simulink model "Inversion"  (Simulink 7.9)
settings: Solver=ode45  StartTime=0.0  StopTime=8  RelTol=1e-3
values from neighbouring files (symbols this model uses):
  g = 9.81    [init.m]
  m = 1.863    [init.m]
undefined symbols (not defined in the file or in its folder): sigbuilder_block
settings Model: Creator=Matthias  LastModifiedBy=Matthias

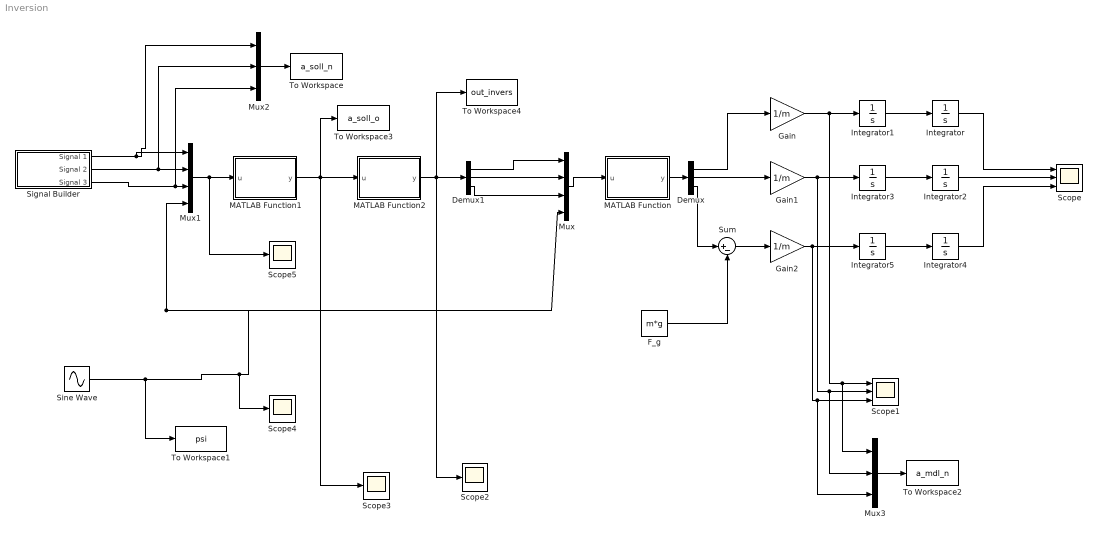
== system Inversion ==
  Demux : Demux  Outputs=3
  Demux1 : Demux  Outputs=3
  F_g : Constant  Value=m*g
  Gain : Gain  Gain=1/m
  Gain1 : Gain  Gain=1/m
  Gain2 : Gain  Gain=1/m
  Integrator{,1..5} (6 alike) : Integrator
  MATLAB Function : MATLAB Function  TreatAsAtomicUnit=on
  MATLAB Function1 : MATLAB Function  TreatAsAtomicUnit=on
  MATLAB Function2 : MATLAB Function  TreatAsAtomicUnit=on
  Mux : Mux
  Mux1 : Mux
  Mux2 : Mux  Inputs=3
  Mux3 : Mux  Inputs=3
  Scope : Scope  NumInputPorts=3
      settings: YMin=-5~-5~-5  YMax=5~5~5
  Scope1 : Scope  NumInputPorts=3
      settings: YMin=-5~-5~-5  YMax=5~5~5
  Scope{2..5} (4 alike) : Scope
      Scope2 settings: SaveName=ScopeData2
      Scope3 settings: SaveName=ScopeData3
      Scope4 settings: SaveName=ScopeData4
      Scope5 settings: SaveName=ScopeData5
  Signal Builder : Subsystem  Tag=STV Subsys  LoadFcn=sigbuilder_block('load',[403.5 141 550.5 395.25 ]);  StartFcn=sigbuilder_block('start');  StopFcn=sigbuilder_block('stop');  ClipboardFcn=sigbuilder_block('clipboard');  mask(Sigbuilder block){}
      mask help: Simulink:masks:SigbuilderBlock_MD
      mask init:
      | if ~strcmp(get_param(bdroot(gcbh),'SimulationStatus'),'stopped') tuvar = sigbuilder_block('maskInit'); end
      settings: CopyFcn=sigbuilder_block('copy');  DeleteFcn=sigbuilder_block('delete');  ModelCloseFcn=sigbuilder_block('modelClose');  PreSaveFcn=sigbuilder_block('preSave');  PauseFcn=sigbuilder_block('pause');  ContinueFcn=sigbuilder_block('continue');  NameChangeFcn=sigbuilder_block('namechange');  OpenFcn=sigbuilder_block('open',[437.6 199.2 550.4 400 ]);  CloseFcn=sigbuilder_block('close');
      mask Display: plot(0, 0, 100, 100,[2, 2, 32, 32, 2], [68, 8, 8, 68, 68],[32, 2], [38, 38], [32, 19, 2],[53, 60, 44], [32, 17, 17, 2],[16, 16, 31, 31]);txt = getActiveGroup(gcbh);text(2, 100, txt,'verticalAlignment', 'top');
  Sine Wave : Sin  SampleTime=0
  Sum : Sum  Inputs=|+-
  To Workspace : ToWorkspace  VariableName=a_soll_n  SampleTime=-1  SaveFormat=Structure With Time
  To Workspace1 : ToWorkspace  VariableName=psi  SampleTime=-1  SaveFormat=Structure With Time
  To Workspace2 : ToWorkspace  VariableName=a_mdl_n  SampleTime=-1  SaveFormat=Structure With Time
  To Workspace3 : ToWorkspace  VariableName=a_soll_o  SampleTime=-1  SaveFormat=Structure With Time
  To Workspace4 : ToWorkspace  VariableName=out_invers  SampleTime=-1  SaveFormat=Structure With Time
  wires:
  Integrator5/1 -> Integrator4/1
  Integrator3/1 -> Integrator2/1
  Integrator1/1 -> Integrator/1
  Integrator/1 -> Scope/1
  Integrator2/1 -> Scope/2
  Integrator4/1 -> Scope/3
  Gain/1 -> Integrator1/1, Scope1/1, Mux3/1
  Gain1/1 -> Integrator3/1, Scope1/2, Mux3/2
  Gain2/1 -> Integrator5/1, Scope1/3, Mux3/3
  Mux/1 -> MATLAB Function/1(u)
  MATLAB Function/1(y) -> Demux/1
  Demux/1 -> Gain/1
  Demux/2 -> Gain1/1
  Mux1/1 -> MATLAB Function1/1(u), Scope5/1
  Sine Wave/1 -> Mux1/4, Mux/4, Scope4/1, To Workspace1/1
  MATLAB Function1/1(y) -> MATLAB Function2/1(u), Scope3/1, To Workspace3/1
  MATLAB Function2/1(y) -> Demux1/1, Scope2/1, To Workspace4/1
  Demux1/1 -> Mux/1
  Demux1/2 -> Mux/2
  Demux1/3 -> Mux/3
  Demux/3 -> Sum/1
  F_g/1 -> Sum/2
  Sum/1 -> Gain2/1
  Signal Builder/1(Signal 1) -> Mux1/1, Mux2/1
  Signal Builder/2(Signal 2) -> Mux1/2, Mux2/2
  Signal Builder/3(Signal 3) -> Mux1/3, Mux2/3
  Mux2/1 -> To Workspace/1
  Mux3/1 -> To Workspace2/1

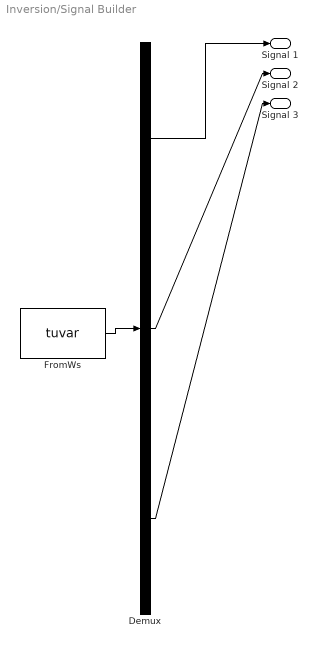
== system Inversion/Signal Builder ==
  Demux : Demux  Tag=STV Demux  Outputs=3
  FromWs : FromWorkspace  Tag=STV FromWs  VariableName=tuvar  SampleTime=0  SigBuilderData=DataTag0  VnvData=DataTag1
      SigBuilderData=|
      | common.afterFinalStr = 'Extrapolate'
      | common.sampleTime = 0
      | dataSet.timeRange = [0 10]
      | dataSet.name = 'Group 1'
      | sbobj.Groups.Name = 'Group 1'
      | sbobj.Groups.Signals(1).Name = 'Signal 1'
      | sbobj.Groups.Signals(1).XData = [0 1.02 1.3 3 7 10]
      | sbobj.Groups.Signals(1).YData = [0 0 -3 2 0 0]
      | sbobj.Groups.Signals(2).Name = 'Signal 2'
      | sbobj.Groups.Signals(2).XData = [0 2 3.4 4.2 6 10]
      | sbobj.Groups.Signals(2).YData = [0 0 5 2 0 0]
      | sbobj.Groups.Signals(3).Name = 'Signal 3'
      | sbobj.Groups.Signals(3).XData = [0 1.48 2 3 5 10]
      | sbobj.Groups.Signals(3).YData = [0 0 1 -1 0 0]
  Signal 1 : Outport  Tag=STV Outport
  Signal 2 : Outport  Tag=STV Outport  Port=2
  Signal 3 : Outport  Tag=STV Outport  Port=3
  wires:
  Demux/1 -> Signal 1/1
  FromWs/1 -> Demux/1
  Demux/2 -> Signal 2/1
  Demux/3 -> Signal 3/1

== matlab function MATLAB Function1 ==
  data: u input double; y output double
function y = fcn(u)
a_nx = u(1);
a_ny = u(2);
a_nz = u(3);
psi  = u(4);

Mz = [cos(psi) sin(psi) 0; -sin(psi) cos(psi) 0; 0 0 1;];
y = Mz * [a_nx;a_ny;a_nz];

== matlab function MATLAB Function ==
  data: u input double; y output double
function y = fcn(u)
T       = u(1);
phi     = u(2);
theta   = u(3);
psi     = u(4);

Mt = [cos(theta) * cos(psi) sin(phi) * sin(theta) * cos(psi) - cos(phi) * sin(psi) cos(phi) * sin(theta) * cos(psi) + sin(phi) * sin(psi); cos(theta) * sin(psi) sin(phi) * sin(theta) * sin(psi) + cos(phi) * cos(psi) cos(phi) * sin(theta) * sin(psi) - sin(phi) * cos(psi); -sin(theta) sin(phi) * cos(theta) cos(phi) * cos(theta);];


y = Mt * [0; 0; T];

== matlab function MATLAB Function2 ==
  data: u input double; y output double
function y = fcn(u)
a_ox = u(1);
a_oy = u(2);
a_oz = u(3);
m = 1.863;
g = 9.81;


T       = m*(sqrt(a_ox^2+a_oy^2+(a_oz+g)^2));
phi     = asin(-(a_oy*m)/T);

theta   = atan(a_ox/(a_oz+g));

y = [T;phi;theta];
